simulink model "prob6_subsystem"  (R2020b)
settings: Solver=VariableStepAuto  StartTime=0.0  StopTime=10.0  RelTol=1e-3
settings Model: Creator=Gopinath Murugan  LastModifiedBy=Gopinath Murugan

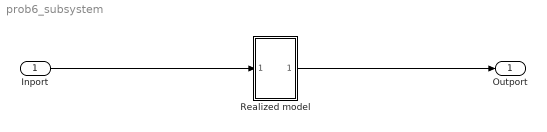
== system prob6_subsystem ==
  Inport : Inport
  Realized model : Subsystem
  Outport : Outport
  wires:
  Inport/1 -> Realized model/1(In1)
  Realized model/1(Out1) -> Outport/1

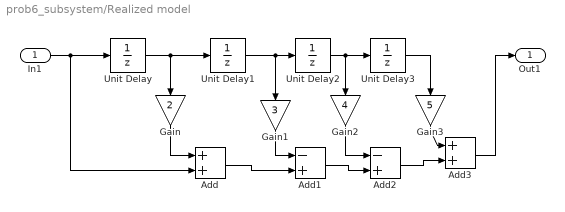
== system prob6_subsystem/Realized model ==
  In1 : Inport
  Add : Sum
  Add1 : Sum  Inputs=-+
  Add2 : Sum  Inputs=-+
  Add3 : Sum
  Gain : Gain  Gain=2
  Gain1 : Gain  Gain=3
  Gain2 : Gain  Gain=4
  Gain3 : Gain  Gain=5
  Unit Delay{,1..3} (4 alike) : UnitDelay  SampleTime=-1  HasFrameUpgradeWarning=on
  Out1 : Outport
  wires:
  Gain1/1 -> Add1/1
  Unit Delay1/1 -> Gain1/1, Unit Delay2/1
  Unit Delay/1 -> Gain/1, Unit Delay1/1
  Gain2/1 -> Add2/1
  Unit Delay2/1 -> Gain2/1, Unit Delay3/1
  Add/1 -> Add1/2
  Add2/1 -> Add3/2
  Gain3/1 -> Add3/1
  Unit Delay3/1 -> Gain3/1
  Add1/1 -> Add2/2
  In1/1 -> Add/2, Unit Delay/1
  Gain/1 -> Add/1
  Add3/1 -> Out1/1
